simulink model "modified_bergman_model"  (R2014a)
settings: Solver=ode3  StartTime=0.0  StopTime=300  FixedStep=0.01  RelTol=1e-3
values from neighbouring files (symbols this model uses):
  D0 = 10    [Modified_Bergman.m]
  drate = 0.05    [Modified_Bergman.m]
  G0 = Gb + p0    (= 276)    [Modified_Bergman.m]    (also in data.m = 287)
  Gb = 81    [Modified_Bergman.m]    (also in data.m = 92)
  I0 = Ib + 396    (= 411)    [Modified_Bergman.m]    (also in data.m = 300)
  Ib = 15    [Modified_Bergman.m]    (also in data.m = 7.3)
  p1 = 0.028735    [Modified_Bergman.m]    (also in data.m = 0.03082)
  p2 = 0.028344    [Modified_Bergman.m]    (also in data.m = 0.02093)
  p3 = 5.035E-5    (= 5.035e-05)    [Modified_Bergman.m]    (also in data.m = 1.06e-05)
  p4 = 0.3    [Modified_Bergman.m]    (also in data.m)
  Rultn = 0.74    [Modified_Bergman.m]
  X0 = 0    [Modified_Bergman.m]    (also in data.m)
libraries: simulink x1
settings Model: Creator=sameer  LastModifiedBy=sameer

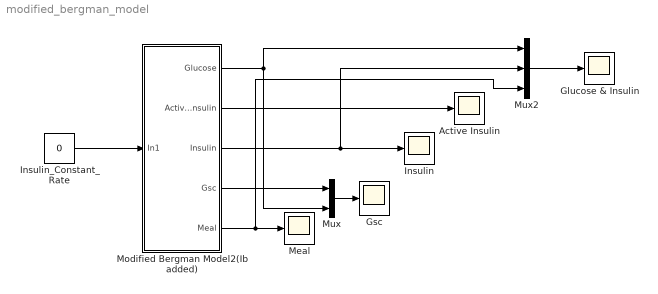
== system modified_bergman_model ==
  Active Insulin : Scope
      settings: ShowLegends=on  SaveName=Active_Insulin
  Glucose & Insulin : Scope
      settings: ShowLegends=on  YMin=275.525  YMax=276  SaveName=Glucose
  Gsc : Scope
      settings: ShowLegends=on  TimeRange=100  SaveName=Gsc
  Insulin : Scope
      settings: ShowLegends=on  SaveName=Insulin
  Insulin_Constant_Rate : Constant  Value=0
  Meal : Scope
      settings: ShowLegends=on  SaveName=Meal
  Modified Bergman Model2(Ib added) : Subsystem
  Mux : Mux  Inputs=2
  Mux2 : Mux  Inputs=3
  wires:
  Modified Bergman Model2(Ib added)/1(Glucose) -> Mux/2, Mux2/1
  Modified Bergman Model2(Ib added)/2(Active Insulin) -> Active Insulin/1
  Modified Bergman Model2(Ib added)/3(Insulin) -> Mux2/2, Insulin/1
  Insulin_Constant_Rate/1 -> Modified Bergman Model2(Ib added)/1(In1)
  Modified Bergman Model2(Ib added)/4(Gsc) -> Mux/1
  Modified Bergman Model2(Ib added)/5(Meal) -> Mux2/3, Meal/1
  Mux/1 -> Gsc/1
  Mux2/1 -> Glucose & Insulin/1

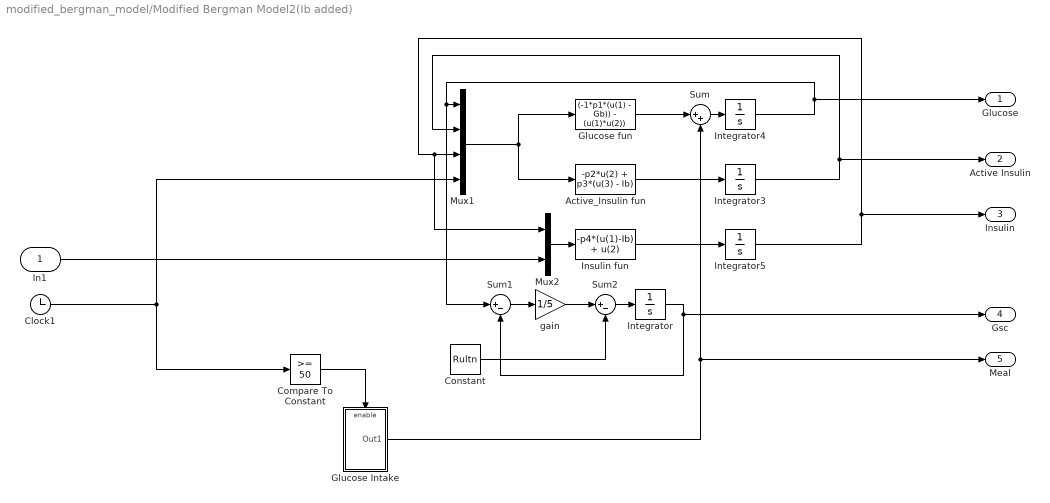
== system modified_bergman_model/Modified Bergman Model2(Ib added) ==
  In1 : Inport
  Active_Insulin fun : Fcn  Expr=-p2*u(2) + p3*(u(3) - Ib)
  Clock1 : Clock
  Compare To Constant : simulink/Logic and Bit Operations/Compare To Constant  relop=>=  const=50  OutDataTypeStr=boolean
  Constant : Constant  Value=Rultn
  Glucose fun : Fcn  Expr=(-1*p1*(u(1) - Gb)) - (u(1)*u(2))
  "Glucose Intake " : Subsystem
  Insulin fun : Fcn  Expr=-p4*(u(1)-Ib) + u(2)
  Integrator : Integrator  InitialCondition=G0 - 5*Rultn
  Integrator3 : Integrator  InitialCondition=X0
  Integrator4 : Integrator  InitialCondition=G0
  Integrator5 : Integrator  InitialCondition=I0
  Mux1 : Mux
  Mux2 : Mux  Inputs=2
  Sum : Sum  Inputs=|++
  Sum1 : Sum  Inputs=|+-
  Sum2 : Sum  Inputs=|+-
  gain : Gain  Gain=1/5
  Glucose : Outport
  Active Insulin : Outport  Port=2
  Insulin : Outport  Port=3
  Gsc : Outport  Port=4
  Meal : Outport  Port=5
  wires:
  gain/1 -> Sum2/1
  Constant/1 -> Sum2/2
  Sum1/1 -> gain/1
  Sum2/1 -> Integrator/1
  Integrator/1 -> Sum1/2, Gsc/1
  In1/1 -> Mux2/2
  Mux2/1 -> Insulin fun/1
  Insulin fun/1 -> Integrator5/1
  "Glucose Intake "/1(Out1) -> Sum/2, Meal/1
  Integrator4/1 -> Glucose/1, Mux1/1, Sum1/1
  Glucose fun/1 -> Sum/1
  Integrator5/1 -> Insulin/1, Mux2/1, Mux1/3
  Mux1/1 -> Active_Insulin fun/1, Glucose fun/1
  Active_Insulin fun/1 -> Integrator3/1
  Sum/1 -> Integrator4/1
  Clock1/1 -> Mux1/4, Compare To Constant/1
  Compare To Constant/1 -> "Glucose Intake "/Enable
  Integrator3/1 -> Active Insulin/1, Mux1/2

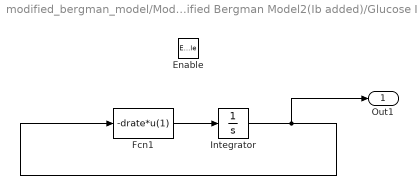
== system modified_bergman_model/Modified Bergman Model2(Ib added)/Glucose Intake  ==
  Enable : EnablePort
  Fcn1 : Fcn  Expr=-drate*u(1)
  Integrator : Integrator  InitialCondition=D0
  Out1 : Outport
  wires:
  Integrator/1 -> Fcn1/1, Out1/1
  Fcn1/1 -> Integrator/1
